simulink subsystem "WindTurbineWithGridAndTransformer"  (R2023b)
settings: Solver=VariableStepAuto  StartTime=0.0  StopTime=10.0  RelTol=1e-3
libraries: simulink x5, ee_lib x4, nesl_utility x4, fl_lib x1
settings Model: Creator=FRESH  LastModifiedBy=FRESH

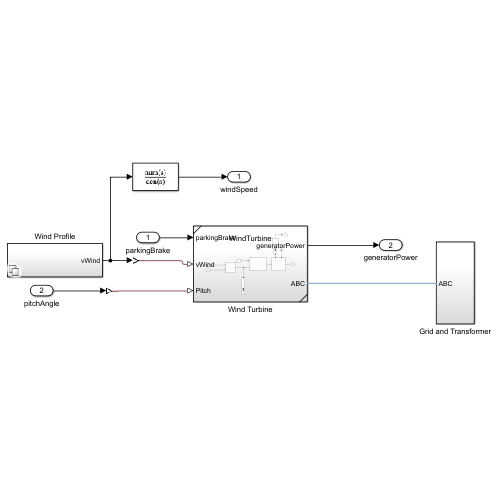
[thumbnail: Simulink's stored preview of the top-level diagram]
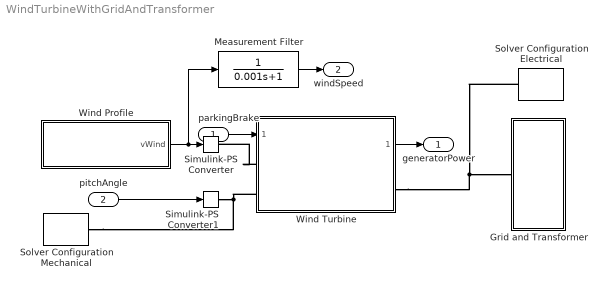
== system WindTurbineWithGridAndTransformer ==
  parkingBrake : Inport
  pitchAngle : Inport  Port=2
  Grid and Transformer : Subsystem
  Measurement Filter : TransferFcn  Denominator=[0.001 1]
  Simulink-PS Converter : nesl_utility/Simulink-PS Converter  PhysicalDomain=network_engine_domain  SubClassName=ps_input  LeftPortType=input  RightPortType=output  PseudoPeriodic=off  Frequencies=[]  NoiseDistribution=none  NoiseParameters=[]  Unit=m/s  AffineConversion=off  FilteringAndDerivatives=filter  SimscapeFilterOrder=1  InputFilterTimeConstant=0.001  UdotUserProvided=0
  Simulink-PS Converter1 : nesl_utility/Simulink-PS Converter  PhysicalDomain=network_engine_domain  SubClassName=ps_input  LeftPortType=input  RightPortType=output  PseudoPeriodic=off  Frequencies=[]  NoiseDistribution=none  NoiseParameters=[]  Unit=deg  AffineConversion=off  FilteringAndDerivatives=filter  SimscapeFilterOrder=1  InputFilterTimeConstant=0.001  UdotUserProvided=0
  Solver Configuration Electrical : nesl_utility/Solver Configuration  PhysicalDomain=network_engine_domain  SubClassName=solver  LeftPortType=input  RightPortType=generic  Tones=[]  Harmonics=[]  SimulateNoise=off  Profile=off  UseLocalSampling=off  EnableSwitchedLinearOptims=on  FrequencyDomain=off  UseCCode=off  RelTol=0.001  AbsTol=0.001  MinStep=1e-09  ToWorkspace=off  RevertToSquareIcSolve=off  NumHomotopyIterations=100  PhasorMode=off  PhasorModeNumHarmonics=1  ConsistencySolver=NEWTON_FTOL  IndexReductionMethod=DerivativeReplacement  DoDC=off  ResidualTolerance=1e-09  ConsistencyTolSource=GLOBAL  ConsistencyAbsTol=0.001  ConsistencyRelTol=0.001  ConsistencyTolFactor=0.001  UseLocalSolver=off  LocalSolverChoice=NE_TRAPEZOIDAL_ADVANCER  ResolveIndetEquations=on  FunctionEvalNumThread=1  LocalSolverSampleTime=1e-5  DoFixedCost=off  MaxNonlinIter=3  MaxModeIter=2  ComputeImpulses=off  ImpulseIterations=2  LinearAlgebra=auto  LinearAlgebraNumThread=0  EquationFormulation=NE_TIME_EF  DelaysMemoryBudget=1024  AutomaticFiltering=on  FilteringTimeConstant=0.001  PartitionStorageMethod=AS_NEEDED  PartitionMemoryBudget=1024  PartitionMethod=ROBUST  MultibodyUseLocalSolver=off  MultibodyLocalSolverChoice=ODE1  MultibodyLocalSolverSampleTime=0.001
  Solver Configuration Mechanical : nesl_utility/Solver Configuration  PhysicalDomain=network_engine_domain  SubClassName=solver  LeftPortType=input  RightPortType=generic  Tones=[]  Harmonics=[]  SimulateNoise=off  Profile=off  UseLocalSampling=off  EnableSwitchedLinearOptims=on  FrequencyDomain=off  UseCCode=off  RelTol=0.001  AbsTol=0.001  MinStep=1e-09  ToWorkspace=off  RevertToSquareIcSolve=off  NumHomotopyIterations=100  PhasorMode=off  PhasorModeNumHarmonics=1  ConsistencySolver=NEWTON_FTOL  IndexReductionMethod=DerivativeReplacement  DoDC=off  ResidualTolerance=1e-09  ConsistencyTolSource=GLOBAL  ConsistencyAbsTol=0.001  ConsistencyRelTol=0.001  ConsistencyTolFactor=0.001  UseLocalSolver=off  LocalSolverChoice=NE_TRAPEZOIDAL_ADVANCER  ResolveIndetEquations=on  FunctionEvalNumThread=1  LocalSolverSampleTime=0.001  DoFixedCost=off  MaxNonlinIter=3  MaxModeIter=2  ComputeImpulses=off  ImpulseIterations=2  LinearAlgebra=auto  LinearAlgebraNumThread=0  EquationFormulation=NE_TIME_EF  DelaysMemoryBudget=1024  AutomaticFiltering=on  FilteringTimeConstant=0.001  PartitionStorageMethod=AS_NEEDED  PartitionMemoryBudget=1024  PartitionMethod=ROBUST  MultibodyUseLocalSolver=off  MultibodyLocalSolverChoice=ODE1  MultibodyLocalSolverSampleTime=0.001
  Wind Profile : Subsystem  Variant=on  VariantControl=Choice
  Wind Turbine : Subsystem  ReferencedSubsystem=WindTurbine
  generatorPower : Outport
  windSpeed : Outport  Port=2
  wires:
  Measurement Filter/1 -> windSpeed/1
  Wind Profile/1(vWind) -> Simulink-PS Converter/1, Measurement Filter/1
  pitchAngle/1 -> Simulink-PS Converter1/1
  parkingBrake/1 -> Wind Turbine/1
  Wind Turbine/1 -> generatorPower/1
  connections:
  Simulink-PS Converter1/RConn1 -- Wind Turbine/LConn2 -- Solver Configuration Mechanical/RConn1
  Wind Turbine/RConn1 -- Grid and Transformer/LConn1 -- Solver Configuration Electrical/RConn1
  Wind Turbine/LConn1 -- Simulink-PS Converter/RConn1

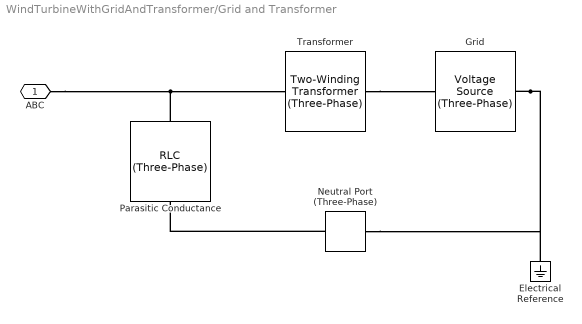
== system WindTurbineWithGridAndTransformer/Grid and Transformer ==
  Electrical Reference : fl_lib/Electrical/Electrical Elements/Electrical Reference
  Grid : ee_lib/Sources/Voltage Source (Three-Phase)  vline_rms=transformerPrimaryVoltage kV  shift=0 deg  freq=gridFrequency Hz  impedance_option=0  SShortCircuit=1e6 A*V  XR=15  R=0.01 Ohm  L=3.97e-4 H  harmonic_option=0  harmonic_orders=[5, 7, 11, 13]  harmonic_ratios=[.1, .1, .1, .1]  G_parasitic=0 1/Ohm  I_specify=off  I_priority=None  I=[0, 0, 0] A  I_nominal_specify=off  I_nominal_unit=A  I_nominal_value=1
  Neutral Port (Three-Phase) : ee_lib/Connectors & References/Neutral Port (Three-Phase)  G_parasitic=1e-12 1/Ohm
      settings: InternalSimscapePortConfiguration="{\"Bottom\":[],\"Left\":[{\"id\":\"N\",\"label\":\"~\",\"type\":\"foundation.electrical.three_phase\"}],\"Right\":[{\"id\":\"n\",\"label\":\"n\",\"type\":\"foundation.electrical.electrical\"}],\"Top\":[]}"
  Parasitic Conductance : ee_lib/Passive/RLC Assemblies/RLC (Three-Phase)  component_structure=ee.enum.rlc.structure.R  R=100000 Ohm  L=1e-3 H  C=1e-6 F  R_parasitic=0 Ohm  G_parasitic=0 1/Ohm  IL_specify=off  IL_priority=High  IL=[0, 0, 0] A  IL_nominal_specify=off  IL_nominal_unit=A  IL_nominal_value=1  VC_specify=off  VC_priority=High  VC=[0, 0, 0] V  VC_nominal_specify=off  VC_nominal_unit=V  VC_nominal_value=1
      settings: InternalSimscapePortConfiguration="{\"Bottom\":[],\"Left\":[{\"id\":\"N1\",\"label\":\"~1\",\"type\":\"foundation.electrical.three_phase\"}],\"Right\":[{\"id\":\"N2\",\"label\":\"~2\",\"type\":\"foundation.electrical.three_phase\"}],\"Top\":[]}"
  Transformer : ee_lib/Passive/Transformers/Two-Winding Transformer (Three-Phase)  SRated=transformerRatedPower MW  FRated=gridFrequency Hz  Winding1Connection=ee.enum.windingconnection.Y  VRated1=transformerPrimaryVoltage kV  Winding2Connection=ee.enum.windingconnection.Y  VRated2=transformerSecondaryVoltage kV  CoreType=ee.enum.coretype.threelimb  pu_Rw1=0.0001  pu_Rw2=0.0001  leakage_reactance_option=ee.enum.transformer_leakage.exclude  pu_Xl1=0.05  pu_Xl2=0.05  magnetizing_resistance_option=ee.enum.transformer_magnetizingResistance.exclude  pu_Rm=500  magnetizing_reactance_option=ee.enum.transformer_magnetizingReactance.exclude  saturation_option=ee.enum.transformer_saturation.exclude  pu_Xm=500  current_data=[0, .002, 1, 2]  magnetic_flux_data=[0, 1.2, 1.5, 1.51]  pu_X0=0.5  i1_specify=off  i1_priority=None  i1=[0, 0, 0] A  i1_nominal_specify=off  i1_nominal_unit=A  i1_nominal_value=1  i2_specify=off  i2_priority=None  i2=[0, 0, 0] A  i2_nominal_specify=off  i2_nominal_unit=A  i2_nominal_value=1  phi_specify=off  phi_priority=None  phi=[0, 0, 0]  phi_nominal_specify=off  phi_nominal_unit=1  phi_nominal_value=1  power_dissipated_specify=off  power_dissipated_priority=None  power_dissipated=0 W  power_dissipated_nominal_specify=off  power_dissipated_nominal_unit=W  power_dissipated_nominal_value=1
      settings: InternalSimscapePortConfiguration="{\"Bottom\":[],\"Left\":[{\"id\":\"N1\",\"label\":\"~1\",\"type\":\"foundation.electrical.three_phase\"}],\"Right\":[{\"id\":\"N2\",\"label\":\"~2\",\"type\":\"foundation.electrical.three_phase\"}],\"Top\":[]}"
  ABC : PMIOPort  Side=Left
  connections:
  Transformer/LConn1 -- Grid/RConn1
  Neutral Port (Three-Phase)/LConn1 -- Parasitic Conductance/RConn1
  Grid/LConn1 -- Electrical Reference/LConn1 -- Neutral Port (Three-Phase)/RConn1
  ABC/RConn1 -- Parasitic Conductance/LConn1 -- Transformer/RConn1

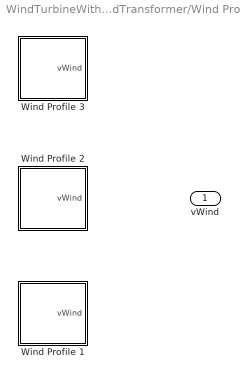
== system WindTurbineWithGridAndTransformer/Wind Profile ==
  Wind Profile 1 : Subsystem  VariantControl=windProfile1
  Wind Profile 2 : Subsystem  VariantControl=windProfile2
  Wind Profile 3 : Subsystem  VariantControl=windProfile3
  vWind : Outport

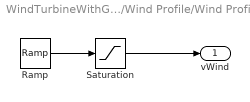
== system WindTurbineWithGridAndTransformer/Wind Profile/Wind Profile 1 ==
  Ramp : simulink/Sources/Ramp  slope=1  start=45  InitialOutput=15
  Saturation : Saturate  UpperLimit=22  LowerLimit=0
  vWind : Outport
  wires:
  Saturation/1 -> vWind/1
  Ramp/1 -> Saturation/1

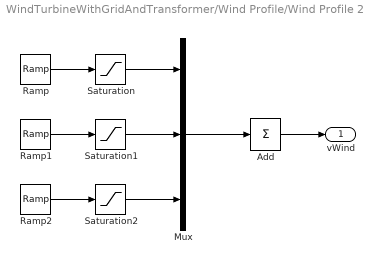
== system WindTurbineWithGridAndTransformer/Wind Profile/Wind Profile 2 ==
  Add : Sum  Inputs=+
  Mux : Mux  Inputs=3
  Ramp : simulink/Sources/Ramp  slope=0.7  start=0  InitialOutput=0
  Ramp1 : simulink/Sources/Ramp  slope=0.7  start=115  InitialOutput=0
  Ramp2 : simulink/Sources/Ramp  slope=-0.7  start=160  InitialOutput=0
  Saturation : Saturate  UpperLimit=10  LowerLimit=0
  Saturation1 : Saturate  UpperLimit=12  LowerLimit=0
  Saturation2 : Saturate  UpperLimit=0  LowerLimit=-7
  vWind : Outport
  wires:
  Saturation2/1 -> Mux/3
  Mux/1 -> Add/1
  Ramp1/1 -> Saturation1/1
  Saturation/1 -> Mux/1
  Add/1 -> vWind/1
  Ramp2/1 -> Saturation2/1
  Ramp/1 -> Saturation/1
  Saturation1/1 -> Mux/2

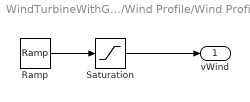
== system WindTurbineWithGridAndTransformer/Wind Profile/Wind Profile 3 ==
  Ramp : simulink/Sources/Ramp  slope=1  start=45  InitialOutput=15
  Saturation : Saturate  UpperLimit=17  LowerLimit=0
  vWind : Outport
  wires:
  Saturation/1 -> vWind/1
  Ramp/1 -> Saturation/1
